simulink model "HvCoorn"  (R2022b)
settings: configuration reference "Icar05FusaMdlCfg" (kept outside this file)
undefined symbols (not defined in the file): BMSActSt_ACChrg, BMSActSt_DCChrg, BMSActSt_disconnect, BMSActSt_offline, BMSActSt_online, BMSActSt_undefined, BMSMainNegRlySt_Clsd_SC, BMSMainNegRlySt_Open_SC, BMSMainNegRlySt_StuckInClsd_SC, BMSMainNegRlySt_StuckInOpen_SC, BMSMainPosRlySt_Clsd_SC, BMSMainPosRlySt_Open_SC, BMSMainPosRlySt_StuckInClsd_SC, BMSPrecRlySt_StuckInOpen_SC, BMSReqSt_ACChrg, BMSReqSt_DCChrg, BMSReqSt_emergencyOffline, BMSReqSt_offline, BMSReqSt_online, Chrg_stCycleBookMod_SC, Chrg_stSingleBookMod_SC, CmpgMod_stInactv_SC, DCDCActSt_buck, DCDCActSt_connected, DCDCActSt_disconnected, DCDCReqSt_buck, DCDCReqSt_standby, EngStrtStop_RefuModDft_SC, EPBActSt_Appld_SC, GearLvr_stDrvGearD_SC, GearLvr_stDrvGearN_SC, GearLvr_stDrvGearP_SC, GearLvr_stDrvGearR_SC, hpp_bACChargeLinkIni_C, hpp_bACChargeLinkOKIni_C, hpp_bAcChgEnaIni_C, hpp_bAcChgPauseIni_C, hpp_bAcLinkTempErrIni_C, hpp_bBattWarmReqIni_C, hpp_bHvilHwErrIni_C, hpp_bHvilStOkIni_C, hpp_bHvRelayClsActIni_C, hpp_bHvRelayOpnActIni_C, hpp_bHvRelayStuckIni_C, hpp_bParked4ChDchgIni_C, hpp_bRemLvBatMntnReqIni_C, hpp_bStartUpReqIni_C, hpp_stHvilCanIni_C, hpp_stWarmTimeCfgRespIni_C, HvCoorn_bAuthEnaSwt_C, HvCoorn_bAuthFailSpdLimOvrd_C, HvCoorn_bAuthFailSpdLimOvrdVal_C, HvCoorn_bAuthStrt_C, HvCoorn_bBMSUnexpdDcnctFailEna_C, HvCoorn_bBuck2RdyBypDCDCEna_C, HvCoorn_bDCChrgFctCfg_C, HvCoorn_bDcChrgWkupEnaChrgLink_C, HvCoorn_bDCDcnct4ACEna_C, HvCoorn_bDCNotBuck2ShtdwnEna_C, HvCoorn_bDrvrLevNotRdyEna_C ... (+295)
libraries: ITKLib x213, simulink x61
(part 7 of 12)

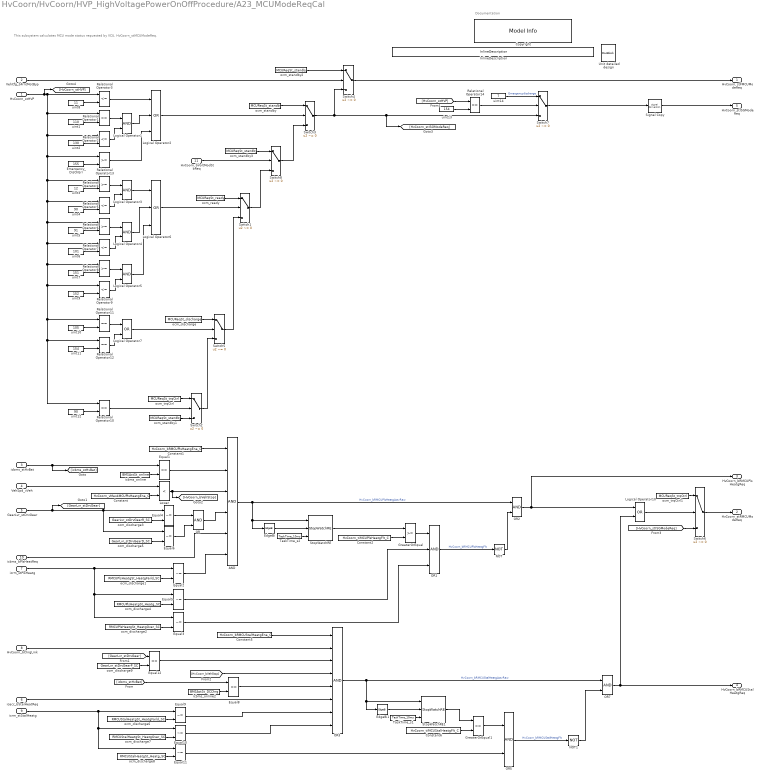
== system HvCoorn/HvCoorn/HVP_HighVoltagePowerOnOffProcedure/A23_MCUModeReqCal ==
  note: This subsystem calculates MCU mode status requested by VCU, HvCoorn_stMCUModeReq.
  note: Documentation
  HvCoorn_stHVP : Inport
  VehCfg_bFrntMotByp : Inport  Port=2
  icbms_stHvBat : Inport  Port=3
  VehSpd_vVeh : Inport  Port=4
  GearLvr_stDrvGear : Inport  Port=5
  icecc_bStalHeatReq : Inport  Port=6
  icrm_stPlsHeatg : Inport  Port=7
  HvCoorn_bChrgLink : Inport  Port=8
  icrm_stStalHeatg : Inport  Port=9
  icbms_bPlsHeatReq : Inport  Port=10
  HvCoorn_bVoltModStbReq : Inport  Port=11
  AND : Logic  Inputs=6  OutDataTypeStr=boolean
  Constant : Constant  Description=[2]  Value=HvCoorn_vMax4MCUPlsHeatgEna_C
      settings: AttributesFormatString=%<Description>
  Constant1 : Constant  Description=[0]  Value=HvCoorn_bRMCUPlsHeatgEna_C
      settings: AttributesFormatString=%<Description>
  Constant2 : Constant  Description=[2]  Value=HvCoorn_tiMCUPlsHeatgFlt_C
      settings: AttributesFormatString=%<Description>
  Constant5 : Constant  Description=[1]  Value=HvCoorn_bRMCUStalHeatgEna_C
      settings: AttributesFormatString=%<Description>
  Constant6 : Constant  Description=[2]  Value=HvCoorn_tiMCUStalHeatgFlt_C
      settings: AttributesFormatString=%<Description>
  Copyright : simulink/Model-Wide Utilities/Model Info  Frame=on  DisplayStringWithTags=|  HorizontalTextAlignment=Left  LeftAlignmentValue=0.02
      | © ITK Engineering Technology (Wu Xi) Co., Ltd. (ITKC)
      | 
      | Model Version: %<ModelVersion>
      | Date: %<LastModificationDate>
  EdgeBi : ITKLib/Memory/EdgeBi  Tag=initial value = 0
      settings: SourceProductName=ITKC_Lib
  EdgeBi1 : ITKLib/Memory/EdgeBi  Tag=initial value = 0
      settings: SourceProductName=ITKC_Lib
  Emergency_DisChErr : Constant  Value=155  OutDataTypeStr=uint8
  Equal1 : RelationalOperator  Operator===  OutDataTypeStr=boolean
  Equal{2..6,9..11} (8 alike) : RelationalOperator  Operator=~=  OutDataTypeStr=boolean
  Equal12 : RelationalOperator  Operator===  OutDataTypeStr=boolean
  Equal8 : RelationalOperator  Operator===  OutDataTypeStr=boolean
  GreaterOrEqual : RelationalOperator  OutDataTypeStr=boolean
  GreaterOrEqual1 : RelationalOperator  OutDataTypeStr=boolean
  InlineDescription : ITKLib/Special/InlineDescription  Tag=HideFromReport  Description=电机模式请求  ShowInLibBrowser=0  RefreshPar=0
      settings: SourceProductName=ITKC_Lib
  Logical Operator{1,3..5} (4 alike) : Logic  AllPortsSameDT=off  OutDataTypeStr=boolean
  Logical Operator10 : Logic  Operator=OR  AllPortsSameDT=off  OutDataTypeStr=boolean
  Logical Operator2 : Logic  Operator=OR  Inputs=3  AllPortsSameDT=off  OutDataTypeStr=boolean
  Logical Operator6 : Logic  Operator=OR  Inputs=3  AllPortsSameDT=off  OutDataTypeStr=boolean
  Logical Operator7 : Logic  Operator=OR  AllPortsSameDT=off  OutDataTypeStr=boolean
  Lower : RelationalOperator  Operator=<  OutDataTypeStr=boolean
  NOT : Logic  Operator=NOT  AllPortsSameDT=off  OutDataTypeStr=boolean
  NOT1 : Logic  Operator=NOT  AllPortsSameDT=off  OutDataTypeStr=boolean
  OR{,2,5,7} (4 alike) : Logic  OutDataTypeStr=boolean
  OR1 : Logic  Inputs=3  OutDataTypeStr=boolean
  OR3 : Logic  Inputs=8  OutDataTypeStr=boolean
  Relational Operator{1,4,6,8,13} (5 alike) : RelationalOperator  OutDataTypeStr=boolean  InputSameDT=off
  Relational Operator{10..12,14} (4 alike) : RelationalOperator  Operator===  OutDataTypeStr=boolean  InputSameDT=off
  Relational Operator{2..3,5,7,9} (5 alike) : RelationalOperator  Operator=<=  OutDataTypeStr=boolean  InputSameDT=off
  Signal Copy : SignalConversion  OverrideOpt=off
  StopWatchRE : ITKLib/TimeCounter/StopWatchRE  Description=""
      settings: SourceProductName=ITKC_Lib
  StopWatchRE1 : ITKLib/TimeCounter/StopWatchRE  Description=""
      settings: SourceProductName=ITKC_Lib
  Switch{1..8} (8 alike) : Switch  Criteria=u2 ~= 0  SaturateOnIntegerOverflow=off  InputSameDT=off
  TaskTime_s1 : Constant  Value=TaskTime_10ms
      settings: AttributesFormatString=[0.01]
  TaskTime_s2 : Constant  Value=TaskTime_10ms
      settings: AttributesFormatString=[0.01]
  Unit detailed design : simulink/Model-Wide Utilities/DocBlock  Tag=HideFromReport  DocumentType=Text
      content=|
      | SMiVCU-3364 - 前后电机模式请求
      | 两驱时，前电机模式请求为0x2:Standby；
      | <高压系统状态>大于等于11，或大于等于110小于等于130，或大于等于155，则<前电机模式请求>为0x2:Standby；否则若<高压系统状态>大于等于12小于等于89，或大于等于91小于等于101，或大于等于151小于等于152，则<前电机模式请求>为0x3:Ready；否则若<高压系统状态>等于105或154，且<前后电机状态>不为0x8：Failure吗，则<前电机模式请求>为0x6:Discharge；否则若<高压系统状态>等于90，则<前电机模式请求>为0x4:TrqCtrl；否则为0x2：Standby。
  icbms_online : Constant  Description=[4]  Value=BMSActSt_online
      settings: AttributesFormatString=[4]
  icbms_online2 : Constant  Description=[8]  Value=BMSActSt_DCChrg
      settings: AttributesFormatString=[8]
  ocm_discharge : Constant  Description=[6]  Value=MCUReqSt_discharge  OutDataTypeStr=uint8
      settings: AttributesFormatString=[6]
  ocm_discharge1 : Constant  Description=[3]  Value=RMCUPlsHeatgSt_HeatgFaild_SC
      settings: AttributesFormatString=%<Description>
  ocm_discharge2 : Constant  Description=[2]  Value=RMCUPlsHeatgSt_HeatgOver_SC
      settings: AttributesFormatString=%<Description>
  ocm_discharge3 : Constant  Description=[5]  Value=GearLvr_stDrvGearR_SC
      settings: AttributesFormatString=%<Description>
  ocm_discharge4 : Constant  Description=[1]  Value=RMCUPlsHeatgSt_Heatg_SC
      settings: AttributesFormatString=%<Description>
  ocm_discharge5 : Constant  Description=[1]  Value=GearLvr_stDrvGearD_SC
      settings: AttributesFormatString=%<Description>
  ocm_discharge6 : Constant  Description=[3]  Value=RMCUStalHeatgSt_HeatgFaild_SC
      settings: AttributesFormatString=%<Description>
  ocm_discharge7 : Constant  Description=[2]  Value=RMCUStalHeatgSt_HeatgOver_SC
      settings: AttributesFormatString=%<Description>
  ocm_discharge8 : Constant  Description=[1]  Value=RMCUStalHeatgSt_Heatg_SC
      settings: AttributesFormatString=%<Description>
  ocm_discharge9 : Constant  Description=[6]  Value=GearLvr_stDrvGearP_SC
      settings: AttributesFormatString=%<Description>
  ocm_ready : Constant  Description=[3]  Value=MCUReqSt_ready  OutDataTypeStr=uint8
      settings: AttributesFormatString=[3]
  ocm_standby{,1..3} (4 alike) : Constant  Description=[2]  Value=MCUReqSt_standby  OutDataTypeStr=uint8
      settings: AttributesFormatString=[2]
  ocm_trqCtrl : Constant  Description=[4]  Value=MCUReqSt_trqCtrl  OutDataTypeStr=uint8
      settings: AttributesFormatString=[4]
  ocm_trqCtrl1 : Constant  Description=[4]  Value=MCUReqSt_trqCtrl  OutDataTypeStr=uint8
      settings: AttributesFormatString=[4]
  uint1 : Constant  Description=Shutdown_DisChErr  Value=110  OutDataTypeStr=uint8
      settings: AttributesFormatString=|
      | %<OutDataTypeStr>
      | %<Description>
  uint10 : Constant  Description=Shutdown_MotDischarge  Value=105  OutDataTypeStr=uint8
      settings: AttributesFormatString=|
      | %<OutDataTypeStr>
      | %<Description>
  uint11 : Constant  Description=Emergency_MotDischarge  Value=154  OutDataTypeStr=uint8
      settings: AttributesFormatString=|
      | %<OutDataTypeStr>
      | %<Description>
  uint12 : Constant  Description=Ready  Value=90  OutDataTypeStr=uint8
      settings: AttributesFormatString=|
      | %<OutDataTypeStr>
      | %<Description>
  uint13 : Constant  Description=Emergency_MotDischarge  Value=154  OutDataTypeStr=uint8
      settings: AttributesFormatString=|
      | %<OutDataTypeStr>
      | %<Description>
  uint14 : Constant  Value=7  OutDataTypeStr=uint8  SampleTime=-1
      settings: AttributesFormatString=%<OutDataTypeStr>
  uint2 : Constant  Description=HcuPowerShutDown  Value=130  OutDataTypeStr=uint8
      settings: AttributesFormatString=|
      | %<OutDataTypeStr>
      | %<Description>
  uint3 : Constant  Description=HvContactorRequest  Value=12  OutDataTypeStr=uint8
      settings: AttributesFormatString=|
      | %<OutDataTypeStr>
      | %<Description>
  uint4 : Constant  Description=SystemReadyWait  Value=90  OutDataTypeStr=uint8
      settings: AttributesFormatString=|
      | %<OutDataTypeStr>
      | %<Description>
  uint5 : Constant  Description=Wait4ComMindChange  Value=91  OutDataTypeStr=uint8
      settings: AttributesFormatString=|
      | %<OutDataTypeStr>
      | %<Description>
  uint6 : Constant  Description=Shutdown_HV  Value=101  OutDataTypeStr=uint8
      settings: AttributesFormatString=|
      | %<OutDataTypeStr>
      | %<Description>
  uint7 : Constant  Description=Emergency_ShutDownIni  Value=151  OutDataTypeStr=uint8
      settings: AttributesFormatString=|
      | %<OutDataTypeStr>
      | %<Description>
  uint8 : Constant  Description=Wait4Communication  Value=11  OutDataTypeStr=uint8
      settings: AttributesFormatString=|
      | %<OutDataTypeStr>
      | %<Description>
  uint9 : Constant  Description=Emergency_ShutdownHV  Value=152  OutDataTypeStr=uint8
      settings: AttributesFormatString=|
      | %<OutDataTypeStr>
      | %<Description>
  HvCoorn_stFMCUModeReq : Outport  VectorParamsAs1DForOutWhenUnconnected=off
  HvCoorn_stRMCUModeReq : Outport  Port=2  VectorParamsAs1DForOutWhenUnconnected=off
  HvCoorn_bRMCUPlsHeatgReq : Outport  Port=3  VectorParamsAs1DForOutWhenUnconnected=off
  HvCoorn_bRMCUStalHeatgReq : Outport  Port=4  VectorParamsAs1DForOutWhenUnconnected=off
  HvCoorn_stISGModeReq : Outport  Port=5  VectorParamsAs1DForOutWhenUnconnected=off
  wires:
  uint8/1 -> Relational Operator3/2
  Switch3/1 -> Switch4/3, Switch7/3, [HvCoorn_stISGModeReq]
  ocm_standby/1 -> Switch3/1
  uint2/1 -> Relational Operator2/2
  uint1/1 -> Relational Operator1/2
  Relational Operator1/1 -> Logical Operator1/1
  Relational Operator2/1 -> Logical Operator1/2
  Logical Operator1/1 -> Logical Operator2/2
  Logical Operator2/1 -> Switch3/2
  uint4/1 -> Relational Operator5/2
  uint3/1 -> Relational Operator4/2
  Relational Operator4/1 -> Logical Operator3/1
  Relational Operator5/1 -> Logical Operator3/2
  ocm_ready/1 -> Switch1/1
  uint6/1 -> Relational Operator7/2
  uint5/1 -> Relational Operator6/2
  Relational Operator6/1 -> Logical Operator4/1
  Relational Operator7/1 -> Logical Operator4/2
  uint9/1 -> Relational Operator9/2
  uint7/1 -> Relational Operator8/2
  Relational Operator8/1 -> Logical Operator5/1
  Relational Operator9/1 -> Logical Operator5/2
  Logical Operator3/1 -> Logical Operator6/1
  Logical Operator4/1 -> Logical Operator6/2
  Logical Operator5/1 -> Logical Operator6/3
  Logical Operator6/1 -> Switch1/2
  uint12/1 -> Relational Operator10/2
  Relational Operator10/1 -> Switch2/2
  uint10/1 -> Relational Operator11/2
  HvCoorn_stHVP/1 -> [HvCoorn_stHVP], Relational Operator10/1, Relational Operator12/1, Relational Operator11/1, Relational Operator9/1, Relational Operator8/1, Relational Operator7/1, Relational Operator6/1, Relational Operator5/1, Relational Operator4/1, Relational Operator13/1, Relational Operator2/1, Relational Operator1/1, Relational Operator3/1
  uint11/1 -> Relational Operator12/2
  Relational Operator11/1 -> Logical Operator7/1
  Relational Operator12/1 -> Logical Operator7/2
  Logical Operator7/1 -> Switch5/2
  ocm_discharge/1 -> Switch5/1
  Switch5/1 -> Switch1/3
  Switch2/1 -> Switch5/3
  ocm_standby1/1 -> Switch2/3
  Emergency_DisChErr/1 -> Relational Operator13/2
  Relational Operator13/1 -> Logical Operator2/3
  ocm_trqCtrl/1 -> Switch2/1
  Switch4/1 -> HvCoorn_stFMCUModeReq/1
  VehCfg_bFrntMotByp/1 -> Switch4/2
  ocm_standby2/1 -> Switch4/1
  icbms_stHvBat/1 -> Equal1/1, [icbms_stHvBat]
  icbms_online/1 -> Equal1/2
  VehSpd_vVeh/1 -> Lower/1
  Constant/1 -> Lower/2
  Equal1/1 -> AND/2
  Lower/1 -> [HvCoorn_bVehStop], AND/3
  ocm_discharge5/1 -> Equal6/2
  Equal4/1 -> OR/1
  ocm_discharge3/1 -> Equal4/2
  Equal6/1 -> OR/2
  GearLvr_stDrvGear/1 -> Equal6/1, Equal4/1, [GearLvr_stDrvGear]
  OR/1 -> AND/4
  icbms_bPlsHeatReq/1 -> AND/5
  ocm_discharge1/1 -> Equal2/2
  icrm_stPlsHeatg/1 -> Equal2/1, Equal3/1, Equal5/1
  Equal2/1 -> AND/6
  AND/1 -> StopWatchRE/1, EdgeBi/1, OR2/1  "HvCoorn_bRMCUPlsHeatgActvRaw"
  Switch6/1 -> HvCoorn_stRMCUModeReq/1
  ocm_trqCtrl1/1 -> Switch6/1
  Constant1/1 -> AND/1
  TaskTime_s2/1 -> StopWatchRE/3
  StopWatchRE/1 -> GreaterOrEqual/1
  Constant2/1 -> GreaterOrEqual/2
  GreaterOrEqual/1 -> OR1/1
  ocm_discharge2/1 -> Equal3/2
  ocm_discharge4/1 -> Equal5/2
  EdgeBi/1 -> StopWatchRE/2
  Equal5/1 -> OR1/2
  Equal3/1 -> OR1/3
  OR1/1 -> NOT/1  "HvCoorn_bRMCUPlsHeatgFlt"
  OR2/1 -> Logical Operator10/1, HvCoorn_bRMCUPlsHeatgReq/1
  NOT/1 -> OR2/2
  [icbms_stHvBat] -> Equal8/1
  icbms_online2/1 -> Equal8/2
  HvCoorn_bChrgLink/1 -> OR3/2
  Equal8/1 -> OR3/5
  icecc_bStalHeatReq/1 -> OR3/6
  Constant5/1 -> OR3/1
  ocm_discharge8/1 -> Equal11/2
  ocm_discharge7/1 -> Equal10/2
  icrm_stStalHeatg/1 -> Equal11/1, Equal10/1, Equal9/1
  ocm_discharge6/1 -> Equal9/2
  Equal9/1 -> OR3/7
  StopWatchRE1/1 -> GreaterOrEqual1/1
  Equal11/1 -> OR5/2
  Constant6/1 -> GreaterOrEqual1/2
  OR5/1 -> NOT1/1  "HvCoorn_bRMCUStalHeatgFlt"
  OR3/1 -> EdgeBi1/1, StopWatchRE1/1, OR7/1  "HvCoorn_bRMCUStalHeatgActvRaw"
  TaskTime_s1/1 -> StopWatchRE1/3
  EdgeBi1/1 -> StopWatchRE1/2
  GreaterOrEqual1/1 -> OR5/1
  Logical Operator10/1 -> Switch6/2
  NOT1/1 -> OR7/2
  OR7/1 -> HvCoorn_bRMCUStalHeatgReq/1, Logical Operator10/2
  [GearLvr_stDrvGear] -> Equal12/1
  ocm_discharge9/1 -> Equal12/2
  Equal12/1 -> OR3/3
  [HvCoorn_bVehStop] -> OR3/4
  Signal Copy/1 -> HvCoorn_stISGModeReq/1
  [HvCoorn_stISGModeReq] -> Switch6/3
  Equal10/1 -> OR3/8
  uint13/1 -> Relational Operator14/2
  Relational Operator3/1 -> Logical Operator2/1
  [HvCoorn_stHVP] -> Relational Operator14/1
  Relational Operator14/1 -> Switch7/2
  Switch7/1 -> Signal Copy/1
  uint14/1 -> Switch7/1  "Emergencydischarge"
  Switch8/1 -> Switch3/3
  Switch1/1 -> Switch8/3
  HvCoorn_bVoltModStbReq/1 -> Switch8/2
  ocm_standby3/1 -> Switch8/1

== system HvCoorn/HvCoorn/HVP_HighVoltagePowerOnOffProcedure/A24_DCDCModeReqCal ==
  note: This subsystem calculates DCDC mode status requested by VCU, HvCoorn_stDCDCModeReq.
  note: Documentation
  HvCoorn_stHVP : Inport
  VehSpd_vVeh : Inport  Port=2
  HvCoorn_bVoltModStbReq : Inport  Port=3
  HvCoorn_stVoltMod : Inport  Port=4
  Abs : Abs
  Calibration2 : Constant  Description=[0.5]  Value=HvCoorn_tiHvOnDCDCBuckDly_C  SampleTime=-1
      settings: AttributesFormatString=%<Description>
  Copyright : simulink/Model-Wide Utilities/Model Info  Frame=on  DisplayStringWithTags=|  HorizontalTextAlignment=Left  LeftAlignmentValue=0.02
      | © ITK Engineering Technology (Wu Xi) Co., Ltd. (ITKC)
      | 
      | Model Version: %<ModelVersion>
      | Date: %<LastModificationDate>
  Equal3 : RelationalOperator  Operator=~=  OutDataTypeStr=boolean
  InlineDescription : ITKLib/Special/InlineDescription  Tag=HideFromReport  Description=DCDC模式请求  ShowInLibBrowser=0  RefreshPar=0
      settings: SourceProductName=ITKC_Lib
  Logical Operator1 : Logic  AllPortsSameDT=off  OutDataTypeStr=boolean
  Logical Operator2 : Logic  Operator=OR  Inputs=3  AllPortsSameDT=off  OutDataTypeStr=boolean
  Logical Operator3 : Logic  Operator=NOT  AllPortsSameDT=off  OutDataTypeStr=boolean
  Logical Operator4 : Logic  AllPortsSameDT=off  OutDataTypeStr=boolean
  Logical Operator5 : Logic  AllPortsSameDT=off  OutDataTypeStr=boolean
  Relational Operator1 : RelationalOperator  Operator===  OutDataTypeStr=boolean  InputSameDT=off
  Relational Operator2 : RelationalOperator  Operator=>  OutDataTypeStr=boolean  InputSameDT=off
  Relational Operator3 : RelationalOperator  Operator=<  OutDataTypeStr=boolean  InputSameDT=off
  Relational Operator6 : RelationalOperator  Operator=>  OutDataTypeStr=boolean  InputSameDT=off
  Switch3 : Switch  Criteria=u2 ~= 0  SaturateOnIntegerOverflow=off  InputSameDT=off
  TaskTime_s2 : Constant  Value=TaskTime_10ms
      settings: AttributesFormatString=[0.01]
  Turn_Off_Delay_Vari : ITKLib/TimeCounter/Turn_Off_Delay_Vari
      settings: AttributesFormatString=TurnOffDelay  SourceProductName=ITKC_Lib
  Unit detailed design : simulink/Model-Wide Utilities/DocBlock  Tag=HideFromReport  DocumentType=Text
      content=|
      | SMiVCU-3365 - DCDC模式请求
      | <高压系统状态>小于17，或<高压系统状态>大于91且<高压系统状态>等于95和<实际车速>的绝对值大于一定值（HvCoorn_v4ShutDown_C，1.5kph）不同时满足，则<DCDC模式请求>为0x1：Standby，否则为0x2：Buck。
  ocdc_buckDcdc : Constant  Description=[2]  Value=DCDCReqSt_buck  OutDataTypeStr=uint8
      settings: AttributesFormatString=[2]
  ocdc_standbyDcdc : Constant  Description=[1]  Value=DCDCReqSt_standby  OutDataTypeStr=uint8
      settings: AttributesFormatString=[1]
  ocm_discharge4 : Constant  Description=[8]  Value=VoltMod_stDCBuck_SC  OutDataTypeStr=uint8
      settings: AttributesFormatString=%<Description>
  sup_vForShutDown_C : Constant  Description=[1.5]  Value=HvCoorn_v4ShutDown_C
      settings: AttributesFormatString=%<Description>
  uint1 : Constant  Description=DCDCBuckReq  Value=17  OutDataTypeStr=uint8
      settings: AttributesFormatString=|
      | %<OutDataTypeStr>
      | %<Description>
  uint2 : Constant  Description=Wait4MindChange  Value=95  OutDataTypeStr=uint8
      settings: AttributesFormatString=|
      | %<OutDataTypeStr>
      | %<Description>
  uint5 : Constant  Description=Wait4ComMindChange  Value=91  OutDataTypeStr=uint8
      settings: AttributesFormatString=|
      | %<OutDataTypeStr>
      | %<Description>
  HvCoorn_stDCDCModeReq : Outport  VectorParamsAs1DForOutWhenUnconnected=off
  wires:
  uint1/1 -> Relational Operator3/2
  HvCoorn_stHVP/1 -> Relational Operator3/1, Relational Operator2/1, Relational Operator1/1
  uint5/1 -> Relational Operator2/2
  Relational Operator2/1 -> Logical Operator4/1
  ocdc_standbyDcdc/1 -> Switch3/1
  Logical Operator2/1 -> Switch3/2
  ocdc_buckDcdc/1 -> Switch3/3
  Switch3/1 -> HvCoorn_stDCDCModeReq/1
  uint2/1 -> Relational Operator1/2
  VehSpd_vVeh/1 -> Abs/1
  sup_vForShutDown_C/1 -> Relational Operator6/2
  Abs/1 -> Relational Operator6/1
  Relational Operator1/1 -> Logical Operator1/1
  Relational Operator6/1 -> Logical Operator1/2
  Logical Operator1/1 -> Logical Operator3/1
  Logical Operator3/1 -> Logical Operator4/2
  Logical Operator4/1 -> Logical Operator2/2
  HvCoorn_bVoltModStbReq/1 -> Logical Operator5/1
  ocm_discharge4/1 -> Equal3/2
  HvCoorn_stVoltMod/1 -> Equal3/1
  Equal3/1 -> Logical Operator5/2
  Logical Operator5/1 -> Logical Operator2/3
  Relational Operator3/1 -> Turn_Off_Delay_Vari/1
  Turn_Off_Delay_Vari/1 -> Logical Operator2/1
  Calibration2/1 -> Turn_Off_Delay_Vari/3
  TaskTime_s2/1 -> Turn_Off_Delay_Vari/2

== system HvCoorn/HvCoorn/HVP_HighVoltagePowerOnOffProcedure/A25_HvilClsReqCal ==
  HvCoorn_stHVP : Inport
  FALSE : Constant  Description=FALSE  Value=0  OutDataTypeStr=boolean
      settings: AttributesFormatString=%<Description>
  Logical Operator1 : Logic  AllPortsSameDT=off  OutDataTypeStr=boolean
  Logical Operator2 : Logic  Operator=OR  AllPortsSameDT=off  OutDataTypeStr=boolean
  Logical Operator3 : Logic  AllPortsSameDT=off  OutDataTypeStr=boolean
  Relational Operator1 : RelationalOperator  Operator=<=  OutDataTypeStr=boolean  InputSameDT=off
  Relational Operator2 : RelationalOperator  Operator=<=  OutDataTypeStr=boolean  InputSameDT=off
  Relational Operator3 : RelationalOperator  OutDataTypeStr=boolean  InputSameDT=off
  Relational Operator4 : RelationalOperator  OutDataTypeStr=boolean  InputSameDT=off
  Relational Operator5 : RelationalOperator  Operator===  OutDataTypeStr=boolean  InputSameDT=off
  Switch1 : Switch  Criteria=u2 ~= 0  SaturateOnIntegerOverflow=off  InputSameDT=off
  Switch3 : Switch  Criteria=u2 ~= 0  SaturateOnIntegerOverflow=off  InputSameDT=off
  TRUE : Constant  Description=TRUE  OutDataTypeStr=boolean
      settings: AttributesFormatString=%<Description>
  Unit Delay2 : UnitDelay  SampleTime=-1  HasFrameUpgradeWarning=on
      settings: AttributesFormatString=<initial=%<X0>>
  WakeUp : Constant  Description=WakeUp  OutDataTypeStr=uint8
      settings: AttributesFormatString=|
      | %<OutDataTypeStr>
      | %<Description>
  WakeUp1 : Constant  Description=Initial_Settings  Value=10  OutDataTypeStr=uint8
      settings: AttributesFormatString=|
      | %<OutDataTypeStr>
      | %<Description>
  WakeUp2 : Constant  Description=NmHoldState  Value=125  OutDataTypeStr=uint8
      settings: AttributesFormatString=|
      | %<OutDataTypeStr>
      | %<Description>
  WakeUp3 : Constant  Description=Emergency_ShutDownIni  Value=151  OutDataTypeStr=uint8
      settings: AttributesFormatString=|
      | %<OutDataTypeStr>
      | %<Description>
  WakeUp4 : Constant  Description=Emergency_NmHoldState  Value=158  OutDataTypeStr=uint8
      settings: AttributesFormatString=|
      | %<OutDataTypeStr>
      | %<Description>
  HvCoorn_bHvilClsReq : Outport  VectorParamsAs1DForOutWhenUnconnected=off
  wires:
  WakeUp1/1 -> Relational Operator3/2
  WakeUp2/1 -> Relational Operator1/2
  Relational Operator3/1 -> Logical Operator1/1
  Relational Operator1/1 -> Logical Operator1/2
  WakeUp3/1 -> Relational Operator4/2
  WakeUp4/1 -> Relational Operator2/2
  Relational Operator4/1 -> Logical Operator3/1
  Relational Operator2/1 -> Logical Operator3/2
  Logical Operator1/1 -> Logical Operator2/1
  Logical Operator3/1 -> Logical Operator2/2
  HvCoorn_stHVP/1 -> Relational Operator3/1, Relational Operator5/1, Relational Operator2/1, Relational Operator4/1, Relational Operator1/1
  WakeUp/1 -> Relational Operator5/2
  TRUE/1 -> Switch3/1
  Logical Operator2/1 -> Switch3/2
  Relational Operator5/1 -> Switch1/2
  Unit Delay2/1 -> Switch1/1
  FALSE/1 -> Switch1/3
  Switch1/1 -> Switch3/3
  Switch3/1 -> Unit Delay2/1, HvCoorn_bHvilClsReq/1

== system HvCoorn/HvCoorn/HVP_HighVoltagePowerOnOffProcedure/A26_DischargeErrCal ==
  note: Documentation
  HvCoorn_stHVP : Inport
  HvCoorn_bStartUpReq : Inport  Port=2
  Copyright : simulink/Model-Wide Utilities/Model Info  Frame=on  DisplayStringWithTags=|  HorizontalTextAlignment=Left  LeftAlignmentValue=0.02
      | © ITK Engineering Technology (Wu Xi) Co., Ltd. (ITKC)
      | 
      | Model Version: %<ModelVersion>
      | Date: %<LastModificationDate>
  EdgeRising1 : ITKLib/Memory/EdgeRising  Tag=initial value = 0
      settings: SourceProductName=ITKC_Lib
  InlineDescription : ITKLib/Special/InlineDescription  Tag=HideFromReport  Description=主动放电故障  ShowInLibBrowser=0  RefreshPar=0
      settings: SourceProductName=ITKC_Lib
  Logical Operator2 : Logic  Operator=OR  AllPortsSameDT=off  OutDataTypeStr=boolean
  RSLatch : ITKLib/Memory/RSLatch
      settings: SourceProductName=ITKC_Lib
  Relational Operator1 : RelationalOperator  Operator===  OutDataTypeStr=boolean  InputSameDT=off
  Relational Operator3 : RelationalOperator  Operator===  OutDataTypeStr=boolean  InputSameDT=off
  Unit detailed design : simulink/Model-Wide Utilities/DocBlock  Tag=HideFromReport  DocumentType=Text
      content=|
      | SMiVCU-3304 - 电压差大使能高压标志位
      | <电池电压>大于<前电机电压>、<DCDC电压>、<OBC电压>、<后电机电压>超过一定值（HvCoorn_uHvDiffOnThrd_C），则激活[电压差大使能高压标志位]
      |
      | SMiVCU-3303 - MCU主动放电完成标志位
      | <前电机主动放电状态反馈>均为0x1：finished，则激活[MCU主动放电完成标志位]。
      |
      | SMiVCU-3308 - 主动放电跳转至关断ECU标志位
      | [高压继电器断开标志位]为1，且以下任一条件满足，则激活[主动放电跳转至关断ECU标志位]：
      | 1.[MCU主动放电完成标志位]为1；
      | 2.<前电机电压>、<DCDC电压>、<OBC电压>、<后电机电压>均小于一定值（HvCoorn_uMax4Shutdown_C，初始值60V）；
      | 3.<状态持续时间>大于一定值（HvCoorn_tiWait4DchaCanLost_C，5s）；
      | 4.[电压差大使能高压标志位]为1，且[上高压失败标志位]为0，且[上高压需求标志位]为1。
      |
      | SMiVCU-3310 - MCU主动放电失败标志位
      | <前电机主动放电状态反馈>均为0x3：Failure（两驱时屏蔽前电机）则激活[MCU主动放电失败标志位]；
      |
      | SMiVCU-3305 - 主动放电跳转至下电Error标志位
      | 以下任一条件满足，则激活[主动放电跳转至下电Error标志位]：
      | 1.<状态持续时间>大于等于一定值（HvCoorn_tiWait4HvDcha_C，初始值120s）；
      | 2.[高压继电器粘连标志位]为1；
      | 3.[MCU主动放电失败标志位]为1；
  uint1 : Constant  Description=Emergency_DisChErr  Value=155  OutDataTypeStr=uint8
      settings: AttributesFormatString=|
      | %<OutDataTypeStr>
      | %<Description>
  uint6 : Constant  Description=Shutdown_DisChErr  Value=110  OutDataTypeStr=uint8
      settings: AttributesFormatString=|
      | %<OutDataTypeStr>
      | %<Description>
  HvCoorn_bActvDischargeErr : Outport  VectorParamsAs1DForOutWhenUnconnected=off
  wires:
  uint6/1 -> Relational Operator3/2
  uint1/1 -> Relational Operator1/2
  Relational Operator3/1 -> Logical Operator2/1
  Relational Operator1/1 -> Logical Operator2/2
  HvCoorn_stHVP/1 -> Relational Operator3/1, Relational Operator1/1
  Logical Operator2/1 -> RSLatch/1
  HvCoorn_bStartUpReq/1 -> EdgeRising1/1
  EdgeRising1/1 -> RSLatch/2
  RSLatch/1 -> HvCoorn_bActvDischargeErr/1

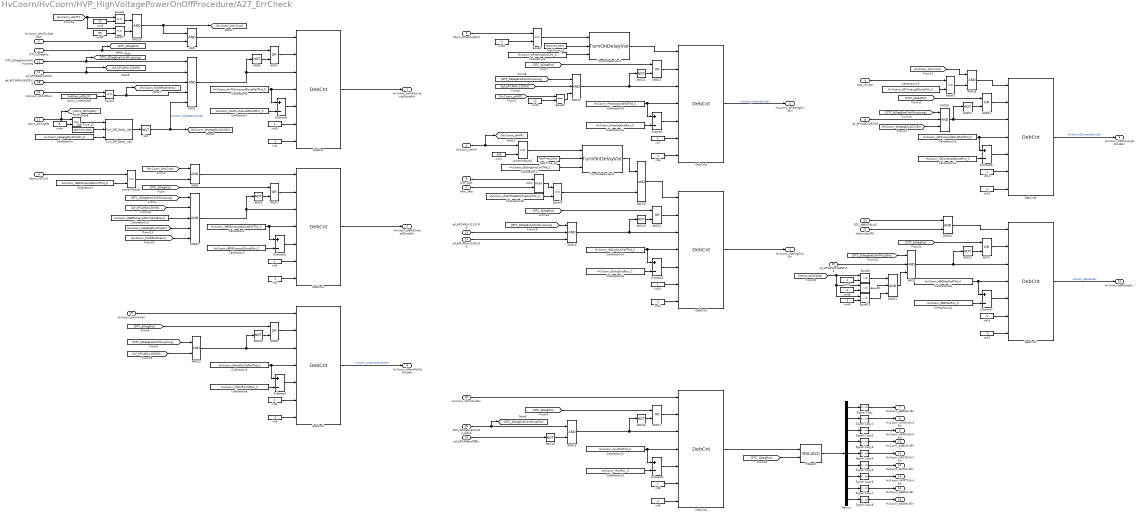
== system HvCoorn/HvCoorn/HVP_HighVoltagePowerOnOffProcedure/A27_ErrCheck ==
  HvCoorn_stHVP : Inport
  DTC_bDiagRst : Inport  Port=2
  icbms_stPrechrgMod : Inport  Port=3
  icbms_uDCLnk : Inport  Port=4
  HvCoorn_bHvRlyOpenAct : Inport  Port=5
  icrm_uAct : Inport  Port=6
  icfm_uAct : Inport  Port=7
  ipf_bPCAN0x353Vld : Inport  Port=8
  icdc_uHvAct : Inport  Port=9
  HvCoorn_bCtrlrHvilErr : Inport  Port=10
  DTC_bDiagEnaCdnWkupLong : Inport  Port=11
  ipf_bPCAN0x130Vld : Inport  Port=12
  ipf_bPCAN0x111S1Vld : Inport  Port=13
  ipf_bPCAN0x110S1Vld : Inport  Port=14
  ipf_bPCANBusOffErr : Inport  Port=15
  DTC_bDiagEnaCdnWkupSho : Inport  Port=16
  icbms_stChrgSts : Inport  Port=17
  ipf_bPCAN0x343S2Vld : Inport  Port=18
  HvCoorn_bHvOnFail : Inport  Port=19
  ipf_bPCAN0x340S1Vld : Inport  Port=20
  icbms_bIsolFlt : Inport  Port=21
  HvCoorn_stVoltMod : Inport  Port=22
  DTC_bBMSFltLvl6 : Inport  Port=23
  AND{,3,15,20,23,28..29,32} (8 alike) : Logic  OutDataTypeStr=boolean
  AND1 : Logic  Inputs=5  OutDataTypeStr=boolean
  AND{4,6,10..11,16,18..19,22,27} (9 alike) : Logic  Operator=NOT  OutDataTypeStr=boolean
  AND{9,12,14,26,31} (5 alike) : Logic  Inputs=3  OutDataTypeStr=boolean
  AND{2,5,7..8,13,17,21,24} (8 alike) : Logic  Operator=OR  OutDataTypeStr=boolean
  AND25 : Logic  Inputs=5  OutDataTypeStr=boolean
  Calibration1 : Constant  Description=[500]  Value=HvCoorn_rBMSUnexpdDcnctFailThd_C  SampleTime=-1
      settings: AttributesFormatString=%<Description>
  Calibration10 : Constant  Description=[5]  Value=HvCoorn_rPrechrgOvtiFailThd_C  SampleTime=-1
      settings: AttributesFormatString=%<Description>
  Calibration11 : Constant  Description=[5]  Value=HvCoorn_rPrechrgOvtiRcv_C  SampleTime=-1
      settings: AttributesFormatString=%<Description>
  Calibration12 : Constant  Description=[50]  Value=HvCoorn_rHvilFailThd_C  SampleTime=-1
      settings: AttributesFormatString=%<Description>
  Calibration13 : Constant  Description=[20]  Value=HvCoorn_rHvilRcv_C  SampleTime=-1
      settings: AttributesFormatString=%<Description>
  Calibration14 : Constant  Description=[5]  Value=HvCoorn_rDchrgOvtiFailThd_C  SampleTime=-1
      settings: AttributesFormatString=%<Description>
  Calibration15 : Constant  Description=[220]  Value=HvCoorn_uDCUnexpdDcnctChk_C  SampleTime=-1
      settings: AttributesFormatString=%<Description>
  Calibration16 : Constant  Description=[5]  Value=HvCoorn_rDchrgOvtiRcv_C  SampleTime=-1
      settings: AttributesFormatString=%<Description>
  Calibration17 : Constant  Description=[3]  Value=HvCoorn_tiDchrgOvtiChkThd_C  SampleTime=-1
      settings: AttributesFormatString=%<Description>
  Calibration18 : Constant  Description=[60]  Value=HvCoorn_uMotThd4DisChrgOvtiChk_C  SampleTime=-1
      settings: AttributesFormatString=%<Description>
  Calibration19 : Constant  Description=[500]  Value=HvCoorn_rDCUnexpdDcnctFailThd_C  SampleTime=-1
      settings: AttributesFormatString=%<Description>
  Calibration2 : Constant  Description=[20]  Value=HvCoorn_rBMSUnexpdDcnctRcv_C  SampleTime=-1
      settings: AttributesFormatString=%<Description>
  Calibration20 : Constant  Description=[0]  Value=HvCoorn_bBMSUnexpdDcnctFailEna_C  SampleTime=-1
      settings: AttributesFormatString=%<Description>
  Calibration21 : Constant  Description=[20]  Value=HvCoorn_rDCUnexpdDcnctRcv_C  SampleTime=-1
      settings: AttributesFormatString=%<Description>
  Calibration23 : Constant  Description=[10]  Value=HvCoorn_rBMSIsoFailThd_C  SampleTime=-1
      settings: AttributesFormatString=%<Description>
  Calibration24 : Constant  Description=[20]  Value=HvCoorn_rBMSIsoRcv_C  SampleTime=-1
      settings: AttributesFormatString=%<Description>
  Calibration3 : Constant  Description=[0]  Value=HvCoorn_uBMSUnexpdDcnctThd_C  SampleTime=-1
      settings: AttributesFormatString=%<Description>
  Calibration4 : Constant  Description=[15]  Value=HvCoorn_tiHeatgDly4ChkErr_C  SampleTime=-1
      settings: AttributesFormatString=%<Description>
  Calibration5 : Constant  Description=[5]  Value=HvCoorn_rMainRlyClsFailThd_C  SampleTime=-1
      settings: AttributesFormatString=%<Description>
  Calibration6 : Constant  Description=[500]  Value=HvCoorn_rHvRlyUnexpdDcnctFailThd_C  SampleTime=-1
      settings: AttributesFormatString=%<Description>
  Calibration7 : Constant  Description=[20]  Value=HvCoorn_rHvRlyUnexpdDcnctRcv_C  SampleTime=-1
      settings: AttributesFormatString=%<Description>
  Calibration8 : Constant  Description=[5]  Value=HvCoorn_rMainRlyClsRcv_C  SampleTime=-1
      settings: AttributesFormatString=%<Description>
  Calibration9 : Constant  Description=[6]  Value=HvCoorn_tiPrechrgOvtiChk_C  SampleTime=-1
      settings: AttributesFormatString=%<Description>
  DebCnt{,1..7} (8 alike) : ITKLib/TimeCounter/DebCnt
      settings: SourceProductName=ITKC_Lib
  Demux : Demux  Outputs=9
  Equal : RelationalOperator  Operator===  OutDataTypeStr=boolean  RndMeth=Simplest  InputSameDT=off
  Equal1 : RelationalOperator  Operator=<=  OutDataTypeStr=boolean
  Equal10 : RelationalOperator  Operator=~=  OutDataTypeStr=boolean  RndMeth=Simplest  InputSameDT=off
  Equal2 : RelationalOperator  Operator===  OutDataTypeStr=boolean
  Equal3 : RelationalOperator  Operator===  OutDataTypeStr=boolean  RndMeth=Simplest  InputSameDT=off
  Equal4 : RelationalOperator  OutDataTypeStr=boolean
  Equal5 : RelationalOperator  Operator===  OutDataTypeStr=boolean  RndMeth=Simplest  InputSameDT=off
  Equal6 : RelationalOperator  OutDataTypeStr=boolean  RndMeth=Simplest  InputSameDT=off
  Equal7 : RelationalOperator  Operator=<=  OutDataTypeStr=boolean  RndMeth=Simplest  InputSameDT=off
  Equal8 : RelationalOperator  Operator=~=  OutDataTypeStr=boolean  RndMeth=Simplest  InputSameDT=off
  Equal9 : RelationalOperator  Operator=~=  OutDataTypeStr=boolean  RndMeth=Simplest  InputSameDT=off
  LowerOrEqual : RelationalOperator  Operator=<=  OutDataTypeStr=boolean
  LowerOrEqual1 : RelationalOperator  Operator===  OutDataTypeStr=boolean
  Min1 : MinMax  Function=max  Inputs=2  InputSameDT=on  SaturateOnIntegerOverflow=on
  Not : Logic  Operator=NOT  AllPortsSameDT=off  OutDataTypeStr=boolean
  RSLatch : ITKLib/Memory/RSLatch
      settings: SourceProductName=ITKC_Lib
  Signal Copy{,1..8} (9 alike) : SignalConversion  OverrideOpt=off
  Subtract{,1..7} (8 alike) : Sum  Inputs=+-  InputSameDT=on  SaturateOnIntegerOverflow=on
  TaskTime_s1 : Constant  Value=TaskTime_10ms
      settings: AttributesFormatString=[0.01]
  TaskTime_s2 : Constant  Value=TaskTime_10ms
      settings: AttributesFormatString=[0.01]
  TaskTime_s3 : Constant  Value=TaskTime_10ms
      settings: AttributesFormatString=[0.01]
  TurnOnDelayVari1 : ITKLib/TimeCounter/TurnOnDelayVari
      settings: AttributesFormatString=TurnOnDelay  SourceProductName=ITKC_Lib
  TurnOnDelayVari2 : ITKLib/TimeCounter/TurnOnDelayVari
      settings: AttributesFormatString=TurnOnDelay  SourceProductName=ITKC_Lib
  Turn_Off_Delay_Vari : ITKLib/TimeCounter/Turn_Off_Delay_Vari
      settings: AttributesFormatString=TurnOffDelay  SourceProductName=ITKC_Lib
  icbms_undefined9 : Constant  Description=[0]  Value=VoltMod_stDft_SC  OutDataTypeStr=uint8
      settings: AttributesFormatString=%<Description>
  int{1..2,4,6,9,11,13,15} (8 alike) : Constant  Value=-1  OutDataTypeStr=int16  SampleTime=-1
      settings: AttributesFormatString=%<OutDataTypeStr>
  int{3,5,7..8,10,12,14,16} (8 alike) : Constant  OutDataTypeStr=int16  SampleTime=-1
      settings: AttributesFormatString=%<OutDataTypeStr>
  uint1 : Constant  Value=105  OutDataTypeStr=uint8  SampleTime=-1
      settings: AttributesFormatString=%<OutDataTypeStr>
  uint2 : Constant  OutDataTypeStr=uint8  SampleTime=-1
      settings: AttributesFormatString=%<OutDataTypeStr>
  uint3 : Constant  Value=12  OutDataTypeStr=uint8  SampleTime=-1
      settings: AttributesFormatString=%<OutDataTypeStr>
  uint4 : Constant  Value=5  OutDataTypeStr=uint8  SampleTime=-1
      settings: AttributesFormatString=%<OutDataTypeStr>
  uint5 : Constant  Value=17  OutDataTypeStr=uint8  SampleTime=-1
      settings: AttributesFormatString=%<OutDataTypeStr>
  uint6 : Constant  Value=95  OutDataTypeStr=uint8  SampleTime=-1
      settings: AttributesFormatString=%<OutDataTypeStr>
  uint7 : Constant  OutDataTypeStr=uint8  SampleTime=-1
      settings: AttributesFormatString=%<OutDataTypeStr>
  uint8 : Constant  Value=2  OutDataTypeStr=uint8  SampleTime=-1
      settings: AttributesFormatString=%<OutDataTypeStr>
  uint9 : Constant  Value=3  OutDataTypeStr=uint8  SampleTime=-1
      settings: AttributesFormatString=%<OutDataTypeStr>
  HvCoorn_bHvRlyUnexpdDcnctErr : Outport  VectorParamsAs1DForOutWhenUnconnected=off
  HvCoorn_bBMSUnexpdDcnctErr : Outport  Port=2  VectorParamsAs1DForOutWhenUnconnected=off
  HvCoorn_bMainRlyFail2ClsErr : Outport  Port=3  VectorParamsAs1DForOutWhenUnconnected=off
  HvCoorn_bPrechrgOvtiErr : Outport  Port=4  VectorParamsAs1DForOutWhenUnconnected=off
  HvCoorn_bDchrgOvtiErr : Outport  Port=5  VectorParamsAs1DForOutWhenUnconnected=off
  HvCoorn_bDCUnexpdDcnctErr : Outport  Port=6  VectorParamsAs1DForOutWhenUnconnected=off
  HvCoorn_bBMSHvilErr : Outport  Port=7  VectorParamsAs1DForOutWhenUnconnected=off
  HvCoorn_bFMCUHvilErr : Outport  Port=8  VectorParamsAs1DForOutWhenUnconnected=off
  HvCoorn_bRMCUHvilErr : Outport  Port=9  VectorParamsAs1DForOutWhenUnconnected=off
  HvCoorn_bOBCHvilErr : Outport  Port=10  VectorParamsAs1DForOutWhenUnconnected=off
  HvCoorn_bDCDCHvilErr : Outport  Port=11  VectorParamsAs1DForOutWhenUnconnected=off
  HvCoorn_bHWHvilErr : Outport  Port=12  VectorParamsAs1DForOutWhenUnconnected=off
  HvCoorn_bWPTCHvilErr : Outport  Port=13  VectorParamsAs1DForOutWhenUnconnected=off
  HvCoorn_bEASHvilErr : Outport  Port=14  VectorParamsAs1DForOutWhenUnconnected=off
  HvCoorn_bBMSIsoErr : Outport  Port=15  VectorParamsAs1DForOutWhenUnconnected=off
  HvCoorn_bISGHvilErr : Outport  Port=16  VectorParamsAs1DForOutWhenUnconnected=off
  wires:
  AND29/1 -> AND/1, [HvCoorn_bHvCnct]
  DebCnt/1 -> HvCoorn_bHvRlyUnexpdDcnctErr/1
  Calibration6/1 -> Subtract1/1, DebCnt/4
  int1/1 -> DebCnt/7
  Subtract1/1 -> DebCnt/5
  int16/1 -> DebCnt/6
  HvCoorn_bHvRlyOpenAct/1 -> AND/2
  AND/1 -> DebCnt/1
  AND1/1 -> AND4/1, DebCnt/3
  AND2/1 -> DebCnt/2
  DTC_bDiagRst/1 -> AND2/1, [DTC_bDiagRst]
  [DTC_bDiagRst] -> AND5/1
  AND5/1 -> DebCnt1/2
  AND25/1 -> DebCnt1/3, AND6/1
  AND3/1 -> DebCnt1/1
  int3/1 -> DebCnt1/6
  Subtract2/1 -> DebCnt1/5
  int2/1 -> DebCnt1/7
  Calibration1/1 -> Subtract2/1, DebCnt1/4
  DebCnt1/1 -> HvCoorn_bBMSUnexpdDcnctErr/1
  [HvCoorn_bHvCnct] -> AND3/1
  AND4/1 -> AND2/2
  AND6/1 -> AND5/2
  LowerOrEqual/1 -> AND3/2
  Calibration3/1 -> LowerOrEqual/2
  icbms_uDCLnk/1 -> LowerOrEqual/1
  AND10/1 -> AND8/2
  DebCnt2/1 -> HvCoorn_bMainRlyFail2ClsErr/1  "HvCoorn_bMainRlyFail2ClsErr"
  Calibration5/1 -> Subtract3/1, DebCnt2/4
  int4/1 -> DebCnt2/7
  Subtract3/1 -> DebCnt2/5
  int5/1 -> DebCnt2/6
  AND23/1 -> AND10/1, DebCnt2/3
  AND8/1 -> DebCnt2/2
  [DTC_bDiagRst] -> AND8/1
  HvCoorn_bHvOnFail/1 -> DebCnt2/1
  TurnOnDelayVari1/1 -> DebCnt3/1
  [DTC_bDiagRst] -> AND13/1
  AND13/1 -> DebCnt3/2
  AND12/1 -> DebCnt3/3, AND11/1
  int7/1 -> DebCnt3/6
  Subtract/1 -> DebCnt3/5
  int6/1 -> DebCnt3/7
  Calibration10/1 -> Subtract/1, DebCnt3/4
  DebCnt3/1 -> HvCoorn_bPrechrgOvtiErr/1  "HvCoorn_bPrechrgOvtiErr"
  AND11/1 -> AND13/2
  Equal2/1 -> TurnOnDelayVari1/1
  uint2/1 -> Equal2/2
  icbms_stPrechrgMod/1 -> Equal2/1
  Calibration9/1 -> TurnOnDelayVari1/3
  TaskTime_s1/1 -> TurnOnDelayVari1/2
  Calibration11/1 -> Subtract/2
  Calibration7/1 -> Subtract1/2
  Calibration2/1 -> Subtract2/2
  Calibration8/1 -> Subtract3/2
  Calibration16/1 -> Subtract5/2
  TaskTime_s3/1 -> TurnOnDelayVari2/2
  Calibration17/1 -> TurnOnDelayVari2/3
  Equal4/1 -> AND20/2
  Calibration18/1 -> Equal4/2
  AND19/1 -> AND21/2
  DebCnt5/1 -> HvCoorn_bDchrgOvtiErr/1
  Calibration14/1 -> DebCnt5/4, Subtract5/1
  Subtract5/1 -> DebCnt5/5
  int10/1 -> DebCnt5/6
  AND14/1 -> AND19/1, DebCnt5/3
  AND21/1 -> DebCnt5/2
  [DTC_bDiagRst] -> AND21/1
  AND20/1 -> DebCnt5/1
  LowerOrEqual1/1 -> TurnOnDelayVari2/1
  Min1/1 -> Equal4/1
  int11/1 -> DebCnt5/7
  icfm_uAct/1 -> Min1/2
  icrm_uAct/1 -> Min1/1
  DTC_bDiagEnaCdnWkupLong/1 -> AND1/1, [DTC_bDiagEnaCdnWkupLong]
  ipf_bPCAN0x130Vld/1 -> AND1/2, [ipf_bPCAN0x130Vld]
  [DTC_bDiagEnaCdnWkupLong] -> AND25/1
  [ipf_bPCAN0x130Vld] -> AND25/2
  [ipf_bPCAN0x130Vld] -> AND23/2
  [DTC_bDiagEnaCdnWkupLong] -> AND23/1
  [ipf_bPCAN0x130Vld] -> AND12/2
  [DTC_bDiagEnaCdnWkupLong] -> AND12/1
  HvCoorn_stHVP/1 -> [HvCoorn_stHVP], LowerOrEqual1/1
  uint1/1 -> LowerOrEqual1/2
  [DTC_bDiagEnaCdnWkupLong] -> AND14/1
  ipf_bPCAN0x111S1Vld/1 -> AND14/2
  ipf_bPCAN0x110S1Vld/1 -> AND14/3
  ipf_bPCANBusOffErr/1 -> AND18/1
  DTC_bDiagEnaCdnWkupSho/1 -> [DTC_bDiagEnaCdnWkupSho], AND15/1
  int9/1 -> DebCnt4/7
  [DTC_bDiagRst] -> AND17/1
  AND17/1 -> DebCnt4/2
  AND15/1 -> DebCnt4/3, AND16/1
  int8/1 -> DebCnt4/6
  Subtract4/1 -> DebCnt4/5
  Calibration12/1 -> Subtract4/1, DebCnt4/4
  AND16/1 -> AND17/2
  Calibration13/1 -> Subtract4/2
  AND18/1 -> AND15/2
  int13/1 -> DebCnt6/7
  AND28/1 -> DebCnt6/1
  AND24/1 -> DebCnt6/2
  AND26/1 -> AND27/1, DebCnt6/3
  int12/1 -> DebCnt6/6
  Subtract6/1 -> DebCnt6/5
  Calibration19/1 -> Subtract6/1, DebCnt6/4
  DebCnt6/1 -> HvCoorn_bDCUnexpdDcnctErr/1  "HvCoorn_bDCUnexpdDcnctErr"
  [DTC_bDiagEnaCdnWkupLong] -> AND26/1
  ipf_bPCAN0x353Vld/1 -> AND26/2
  AND27/1 -> AND24/2
  [DTC_bDiagRst] -> AND24/1
  icdc_uHvAct/1 -> Equal1/1
  Calibration15/1 -> Equal1/2
  Calibration21/1 -> Subtract6/2
  Equal1/1 -> AND28/2
  icbms_stChrgSts/1 -> [icbms_stChrgSts], Equal/1
  uint4/1 -> Equal/2
  ipf_bPCAN0x343S2Vld/1 -> AND1/3
  [HvCoorn_stHVP] -> Equal7/1, Equal6/1
  uint5/1 -> Equal6/2
  Equal6/1 -> AND29/1
  Equal7/1 -> AND29/2
  uint6/1 -> Equal7/2
  [HvCoorn_bHvCnct] -> AND28/1
  uint3/1 -> Equal5/2
  [HvCoorn_stHVP] -> Equal5/1
  Equal5/1 -> AND12/3
  TurnOnDelayVari2/1 -> AND20/1
  Calibration20/1 -> AND25/3
  Not/1 -> AND1/5, [HvCoorn_bHeatgDly4ChkErr]  "HvCoorn_bHeatgDly4ChkErr"
  TaskTime_s2/1 -> Turn_Off_Delay_Vari/2
  Calibration4/1 -> Turn_Off_Delay_Vari/3
  Turn_Off_Delay_Vari/1 -> Not/1
  Equal/1 -> Turn_Off_Delay_Vari/1
  [HvCoorn_bHeatgDly4ChkErr] -> AND25/4
  [HvCoorn_bHeatgDly4ChkErr] -> AND26/3
  HvCoorn_bCtrlrHvilErr/1 -> DebCnt4/1
  RSLatch/1 -> Demux/1
  Demux/1 -> Signal Copy/1
  Demux/2 -> Signal Copy1/1
  Demux/3 -> Signal Copy2/1
  Demux/4 -> Signal Copy3/1
  Demux/5 -> Signal Copy4/1
  Demux/6 -> Signal Copy5/1
  Signal Copy/1 -> HvCoorn_bBMSHvilErr/1
  Signal Copy1/1 -> HvCoorn_bFMCUHvilErr/1
  Signal Copy2/1 -> HvCoorn_bRMCUHvilErr/1
  Signal Copy3/1 -> HvCoorn_bOBCHvilErr/1
  Signal Copy4/1 -> HvCoorn_bDCDCHvilErr/1
  Signal Copy5/1 -> HvCoorn_bHWHvilErr/1
  Signal Copy7/1 -> HvCoorn_bEASHvilErr/1
  Signal Copy6/1 -> HvCoorn_bWPTCHvilErr/1
  Demux/7 -> Signal Copy6/1
  Demux/8 -> Signal Copy7/1
  Subtract7/1 -> DebCnt7/5
  [DTC_bDiagRst] -> AND7/1
  [DTC_bDiagEnaCdnWkupSho] -> AND9/1
  Calibration24/1 -> Subtract7/2
  int15/1 -> DebCnt7/7
  Calibration23/1 -> DebCnt7/4, Subtract7/1
  AND9/1 -> AND22/1, DebCnt7/3
  DebCnt7/1 -> HvCoorn_bBMSIsoErr/1  "HvCoorn_bBMSIsoErr"
  int14/1 -> DebCnt7/6
  ipf_bPCAN0x340S1Vld/1 -> AND9/2
  AND7/1 -> DebCnt7/2
  AND22/1 -> AND7/2
  Signal Copy8/1 -> HvCoorn_bISGHvilErr/1
  Demux/9 -> Signal Copy8/1
  HvCoorn_stVoltMod/1 -> Equal3/1
  icbms_undefined9/1 -> Equal3/2
  Equal3/1 -> AND1/4, [HvCoorn_bVoltModInactv]
  [HvCoorn_bVoltModInactv] -> AND25/5
  uint7/1 -> Equal8/2
  [icbms_stChrgSts] -> Equal9/1, Equal10/1, Equal8/1
  uint8/1 -> Equal9/2
  uint9/1 -> Equal10/2
  Equal8/1 -> AND31/1
  Equal9/1 -> AND31/2
  Equal10/1 -> AND31/3
  AND31/1 -> AND9/3
  icbms_bIsolFlt/1 -> AND32/2
  AND32/1 -> DebCnt7/1
  DTC_bBMSFltLvl6/1 -> AND32/1
  DebCnt4/1 -> RSLatch/1
  [DTC_bDiagRst] -> RSLatch/2

== system HvCoorn/HvCoorn/HVP_HighVoltagePowerOnOffProcedure/A28_V2L ==
  HvCoorn_stHVP : Inport
  icicm_stIvtrSwt : Inport  Port=2
  PwrLimBatt_pwrContnsDChrg : Inport  Port=3
  icobc_bDchrgrCnct : Inport  Port=4
  HvCoorn_bParked4ChDchg : Inport  Port=5
  icbms_pctHVBatSOCDisp : Inport  Port=6
  icicm_pctSOCV2XLimSet : Inport  Port=7
  icobc_stOBCMode : Inport  Port=8
  HvCoorn_bDCChrgLink : Inport  Port=9
  HvCoorn_pctSOCV2XLimSetEER : Inport  Port=10
  icicm_bOTAOn : Inport  Port=11
  EngStrtStop_bFuChrgActvEEW : Inport  Port=12
  icobc_stV2LFltTyp : Inport  Port=13
  AND : Logic  Inputs=8  OutDataTypeStr=boolean
  AND{1..2,4..5} (4 alike) : Logic  OutDataTypeStr=boolean
  AND3 : Logic  Operator=OR  Inputs=11  OutDataTypeStr=boolean
  AND7 : Logic  Operator=OR  OutDataTypeStr=boolean
  Calibration1 : Constant  Description=[6600]  Value=HvCoorn_pwrV2LEnaLowLim_C  SampleTime=-1
      settings: AttributesFormatString=%<Description>
  Calibration2 : Constant  Description=[5]  Value=HvCoorn_tiV2LWaitOBCRsp_C  SampleTime=-1
      settings: AttributesFormatString=%<Description>
  Calibration3 : Constant  Description=[5]  Value=HvCoorn_pctBatSocV2LExThd_C  SampleTime=-1
      settings: AttributesFormatString=%<Description>
  Constant1 : Constant  Description=[3]  Value=OBCActSt_charging
      settings: AttributesFormatString=[3]
  Constant2 : Constant  Description=[9]  Value=OBCActSt_V2LAndV2In
      settings: AttributesFormatString=[9]
  Constant4 : Constant  Description=[7]  Value=OBCActSt_failure
      settings: AttributesFormatString=[7]
  Constant5 : Constant  Description=[4]  Value=OBCActSt_V2L
      settings: AttributesFormatString=[4]
  Constant6 : Constant  Description=[7]  Value=OBCActSt_failure
      settings: AttributesFormatString=[7]
  EdgeRising : ITKLib/Memory/EdgeRising  Tag=initial value = 0
      settings: SourceProductName=ITKC_Lib
  Equal{,1..2,6..7,14..17} (9 alike) : RelationalOperator  Operator===  OutDataTypeStr=boolean  RndMeth=Simplest  InputSameDT=off
  Equal10 : RelationalOperator  OutDataTypeStr=boolean  RndMeth=Simplest  InputSameDT=off
  Equal11 : RelationalOperator  Operator=<=  OutDataTypeStr=boolean  RndMeth=Simplest  InputSameDT=off
  Equal12 : RelationalOperator  OutDataTypeStr=boolean  RndMeth=Simplest  InputSameDT=off
  Equal13 : RelationalOperator  Operator=<  OutDataTypeStr=boolean  RndMeth=Simplest  InputSameDT=off
  Equal3 : RelationalOperator  OutDataTypeStr=boolean  RndMeth=Simplest  InputSameDT=off
  Equal4 : RelationalOperator  Operator=~=  OutDataTypeStr=boolean  RndMeth=Simplest  InputSameDT=off
  Equal5 : RelationalOperator  Operator=>  OutDataTypeStr=boolean  RndMeth=Simplest  InputSameDT=off
  Equal8 : RelationalOperator  Operator=~=  OutDataTypeStr=boolean  RndMeth=Simplest  InputSameDT=off
  Equal9 : RelationalOperator  Operator=<=  OutDataTypeStr=boolean  RndMeth=Simplest  InputSameDT=off
  Not{,1..7} (8 alike) : Logic  Operator=NOT  AllPortsSameDT=off  OutDataTypeStr=boolean
  OR : Logic  OutDataTypeStr=boolean
  OR1 : Logic  Operator=OR  Inputs=3  OutDataTypeStr=boolean
  RSLatch : ITKLib/Memory/RSLatch
      settings: SourceProductName=ITKC_Lib
  RSLatch1 : ITKLib/Memory/RSLatch
      settings: SourceProductName=ITKC_Lib
  Signal Copy : SignalConversion  OverrideOpt=off
  Switch{,1..3} (4 alike) : Switch  Criteria=u2 ~= 0  SaturateOnIntegerOverflow=off  InputSameDT=off
      settings: AttributesFormatString=Criteria : %<Criteria>
  TRUE : Constant  Description=TRUE  OutDataTypeStr=boolean  SampleTime=-1
      settings: AttributesFormatString=%<Description>
  TaskTime_s2 : Constant  Value=TaskTime_10ms
      settings: AttributesFormatString=[0.01]
  TurnOnDelayVari : ITKLib/TimeCounter/TurnOnDelayVari
      settings: AttributesFormatString=TurnOnDelay  SourceProductName=ITKC_Lib
  Unit Delay : UnitDelay  SampleTime=-1  HasFrameUpgradeWarning=on
      settings: AttributesFormatString=<initial=%<x0>>
  uint1 : Constant  Value=2  OutDataTypeStr=uint8  SampleTime=-1
      settings: AttributesFormatString=%<OutDataTypeStr>
  uint10 : Constant  Value=2  OutDataTypeStr=uint8  SampleTime=-1
      settings: AttributesFormatString=%<OutDataTypeStr>
  uint11 : Constant  Value=3  OutDataTypeStr=uint8  SampleTime=-1
      settings: AttributesFormatString=%<OutDataTypeStr>
  uint2 : Constant  OutDataTypeStr=uint8  SampleTime=-1
      settings: AttributesFormatString=%<OutDataTypeStr>
  uint3 : Constant  Value=20  OutDataTypeStr=uint8  SampleTime=-1
      settings: AttributesFormatString=%<OutDataTypeStr>
  uint4 : Constant  Value=100  OutDataTypeStr=uint8  SampleTime=-1
      settings: AttributesFormatString=%<OutDataTypeStr>
  uint5 : Constant  Description=[20]  Value=HvCoorn_pctSOCV2XLimSetDft_C  SampleTime=-1
      settings: AttributesFormatString=%<Description>
  uint6 : Constant  Value=20  OutDataTypeStr=uint8  SampleTime=-1
      settings: AttributesFormatString=%<OutDataTypeStr>
  uint7 : Constant  Value=100  OutDataTypeStr=uint8  SampleTime=-1
      settings: AttributesFormatString=%<OutDataTypeStr>
  uint8 : Constant  Value=89  OutDataTypeStr=uint8  SampleTime=-1
      settings: AttributesFormatString=%<OutDataTypeStr>
  uint9 : Constant  OutDataTypeStr=uint8  SampleTime=-1
      settings: AttributesFormatString=%<OutDataTypeStr>
  HvCoorn_bV2LReq : Outport  VectorParamsAs1DForOutWhenUnconnected=off
  HvCoorn_bV2LActv : Outport  Port=2  VectorParamsAs1DForOutWhenUnconnected=off
  HvCoorn_pctSOCV2XLimSetEEW : Outport  Port=3  VectorParamsAs1DForOutWhenUnconnected=off
  wires:
  HvCoorn_stHVP/1 -> Equal/1
  uint8/1 -> Equal/2
  icicm_stIvtrSwt/1 -> [icicm_stIvtrSwt], Equal1/1
  uint1/1 -> Equal1/2  "enable"
  Equal1/1 -> AND/2
  uint2/1 -> Equal2/2  "disable"
  PwrLimBatt_pwrContnsDChrg/1 -> Equal3/1
  Calibration1/1 -> Equal3/2
  icobc_bDchrgrCnct/1 -> [icobc_bDchrgrCnct], Not3/1, AND/4
  icobc_stOBCMode/1 -> Equal4/1, [icobc_stOBCMode], Equal8/1
  HvCoorn_bDCChrgLink/1 -> Not/1, AND3/7
  Equal/1 -> AND/1, Not5/1
  Equal3/1 -> AND/3, Not2/1
  HvCoorn_bParked4ChDchg/1 -> AND/5, Not4/1
  Switch2/1 -> AND/6, Not7/1
  OR/1 -> AND/7
  Not/1 -> AND/8
  AND/1 -> RSLatch/1  "HvCoorn_bV2LReqSet"
  RSLatch/1 -> AND2/1, HvCoorn_bV2LReq/1, TurnOnDelayVari/1
  [icobc_stOBCMode] -> Equal6/1
  Constant5/1 -> Equal6/2
  AND1/1 -> Unit Delay/1
  Unit Delay/1 -> AND3/11  "HvCoorn_bV2LReqOvtiRst"
  AND2/1 -> HvCoorn_bV2LActv/1
  Not1/1 -> AND1/1
  TurnOnDelayVari/1 -> AND1/2
  [icicm_stIvtrSwt] -> Equal2/1
  Equal2/1 -> EdgeRising/1
  Not5/1 -> AND3/1
  EdgeRising/1 -> AND3/2
  Not2/1 -> AND3/3
  Not3/1 -> AND3/4
  Not4/1 -> AND3/5
  [icobc_stOBCMode] -> Equal7/1
  Constant4/1 -> Equal7/2
  Equal7/1 -> AND3/8
  AND3/1 -> RSLatch/2  "HvCoorn_bV2LReqRst"
  TaskTime_s2/1 -> TurnOnDelayVari/2
  Calibration2/1 -> TurnOnDelayVari/3
  HvCoorn_pctSOCV2XLimSetEER/1 -> Signal Copy/1
  Switch1/1 -> [HvCoorn_pctSOCV2XLimSetEEW], HvCoorn_pctSOCV2XLimSetEEW/1
  Signal Copy/1 -> Switch/1, Equal10/1, Equal9/1  "HvCoorn_pctSOCV2XLimSetEER"
  Switch/1 -> Switch1/3
  AND5/1 -> Switch1/2
  Equal11/1 -> AND5/1
  uint4/1 -> Equal11/2
  icicm_pctSOCV2XLimSet/1 -> Equal11/1, Equal12/1, Switch1/1
  uint3/1 -> Equal12/2
  Equal12/1 -> AND5/2
  AND4/1 -> Switch/2
  Equal10/1 -> AND4/2
  uint6/1 -> Equal10/2
  uint7/1 -> Equal9/2
  Equal9/1 -> AND4/1
  uint5/1 -> Switch/3
  [HvCoorn_pctSOCV2XLimSetEEW] -> Equal5/2
  icbms_pctHVBatSOCDisp/1 -> [icbms_pctHVBatSOCDisp], Equal5/1
  icicm_bOTAOn/1 -> AND3/9
  Equal5/1 -> Switch2/3
  EngStrtStop_bFuChrgActvEEW/1 -> [EngStrtStop_bFuChrgActvEEW], Switch2/2
  TRUE/1 -> Switch2/1
  Switch3/1 -> AND3/6
  [icbms_pctHVBatSOCDisp] -> Equal13/1
  Calibration3/1 -> Equal13/2
  Not7/1 -> Switch3/3
  Equal13/1 -> Switch3/1
  [EngStrtStop_bFuChrgActvEEW] -> Switch3/2
  Constant2/1 -> Equal14/2
  Equal14/1 -> AND7/2
  [icobc_stOBCMode] -> Equal14/1
  Equal6/1 -> AND7/1
  AND7/1 -> Not1/1, AND2/2
  Constant1/1 -> Equal4/2
  Constant6/1 -> Equal8/2
  Equal4/1 -> OR/1
  Equal8/1 -> OR/2
  icobc_stV2LFltTyp/1 -> Equal16/1, Equal17/1, Equal15/1
  uint9/1 -> Equal15/2
  uint10/1 -> Equal16/2
  uint11/1 -> Equal17/2
  Equal15/1 -> OR1/1
  Equal16/1 -> OR1/2
  Equal17/1 -> OR1/3
  OR1/1 -> RSLatch1/1
  RSLatch1/1 -> AND3/10
  [icobc_bDchrgrCnct] -> Not6/1
  Not6/1 -> RSLatch1/2
